simulink model "tests"  (R2015a)
settings: Solver=ode45  StartTime=0.0  StopTime=10.0  RelTol=1e-3
libraries: simulink x4
settings Model: Creator=shizue  LastModifiedBy=shizue

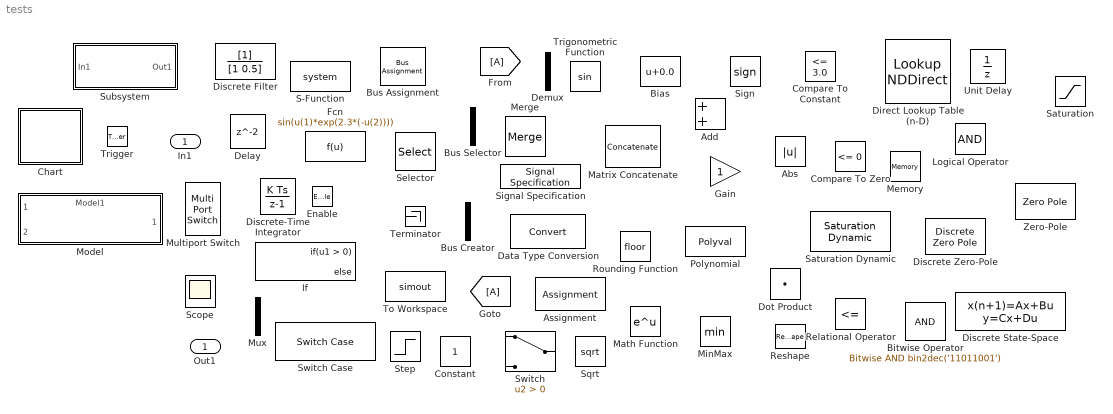
== system tests ==
  In1 : Inport
  Enable : EnablePort
  Trigger : TriggerPort  PortDimensions=1
  Abs : Abs
  Add : Sum
  Assignment : Assignment  DiagnosticForDimensions=Warning
  Bias : Bias  Bias=0.0
  Bitwise Operator : simulink/Logic and Bit Operations/Bitwise Operator  logicop=AND  UseBitMask=on  BitMask=bin2dec('11011001')  BitMaskRealWorld=Stored Integer
  Bus Assignment : BusAssignment
  Bus Creator : BusCreator  Inputs=2
  Bus Selector : BusSelector  OutputSignals=signal1,signal2
  Chart : Stateflow chart  TreatAsAtomicUnit=on
  Compare To Constant : simulink/Logic and Bit Operations/Compare To Constant  relop=<=  const=3.0  OutDataTypeStr=boolean
  Compare To Zero : simulink/Logic and Bit Operations/Compare To Zero  relop=<=  OutDataTypeStr=boolean
  Constant : Constant
  Data Type Conversion : DataTypeConversion
  Delay : Delay
  Demux : Demux  Outputs=2
  Direct Lookup Table (n-D) : LookupNDDirect
  Discrete Zero-Pole : DiscreteZeroPole  Poles=[0 0.5]  Gain=1
  Discrete Filter : DiscreteFilter
  Discrete State-Space : DiscreteStateSpace
  Discrete-Time Integrator : DiscreteIntegrator  InitialConditionSetting=State (most efficient)
  Dot Product : DotProduct  InputSameDT=on  OutDataTypeStr=Inherit: Inherit via internal rule
  Fcn : Fcn  Expr=sin(u(1)*exp(2.3*(-u(2))))
  Gain : Gain
  If : If
  Logical Operator : Logic  AllPortsSameDT=off  OutDataTypeStr=boolean
  Math Function : Math  SaturateOnIntegerOverflow=on
  Matrix Concatenate : Concatenate  Mode=Multidimensional array  ConcatenateDimension=2
  Memory : Memory
  Merge : Merge
  MinMax : MinMax
  Model : ModelReference  ModelNameDialog=Model1.slx  SimulationMode=Normal  ModelReferenceVersion=1.2  CopyOfModelName=Model1.slx  DefaultDataLogging=on
  Multiport Switch : MultiPortSwitch
  Mux : Mux  Inputs=2
  Polynomial : Polyval  Coefs=[ +2.081618890e-019, -1.441693666e-014, +4.719686976e-010, -8.536869453e-006, +1.621573104e-001, -8.087801117e+001 ]
  Relational Operator : RelationalOperator  Operator=<=  OutDataTypeStr=boolean
  Reshape : Reshape
  Rounding Function : Rounding
  S-Function : S-Function
  Saturation : Saturate
  Saturation Dynamic : simulink/Discontinuities/Saturation Dynamic  OutMin=[]  OutMax=[]  OutDataTypeStr=Inherit: Same as second input  OutDataType=fixdt(1, 16)  OutScaling=2^-10  DoSatur=off
  Scope : Scope
  Selector : Selector  InputPortWidth=3  Indices=[1 3]
  Sign : Signum
  Signal Specification : SignalSpecification
  Sqrt : Sqrt  SaturateOnIntegerOverflow=on
  Step : Step  SampleTime=0
  Subsystem : Subsystem
  Switch : Switch  Criteria=u2 > Threshold
  Switch Case : SwitchCase
  Terminator : Terminator
  To Workspace : ToWorkspace  VariableName=simout  SaveFormat=Timeseries  SampleTime=-1
  Trigonometric Function : Trigonometry
  Unit Delay : UnitDelay  SampleTime=-1
  Zero-Pole : ZeroPole  Poles=[0 -1]
  Out1 : Outport

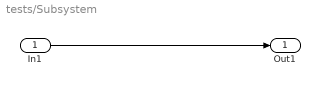
== system tests/Subsystem ==
  In1 : Inport
  Out1 : Outport
  wires:
  In1/1 -> Out1/1

== stateflow chart tests/Chart ==
